simulink model "testRemoteVelEnc"  (Simulink 7.3)
settings: Solver=ode45  SolverMode=SingleTasking  StartTime=0.0  StopTime=inf  FixedStep=0.5  RelTol=1e-3  AbsTol=1e-6
libraries: utility x1
settings Model: Creator=dmedonza  LastModifiedBy=yo
settings DataIOCC: SaveOutput=off  SignalLogging=off  SaveTime=off
settings OptimizationCC: BooleanDataType=off
settings DebuggingCC: SaveWithParameterizedLinksMsg=none  SignalResolutionControl=TryResolveAllWithWarning  SolverPrmCheckMsg=none  MultiTaskDSMMsg=warning  MultiTaskCondExecSysMsg=none  StrictBusMsg=None
settings HardwareCC: TargetUnknown=on
settings RTWCC: TemplateMakefile=grt_vc.tmf  IncludeERTFirstTime=on

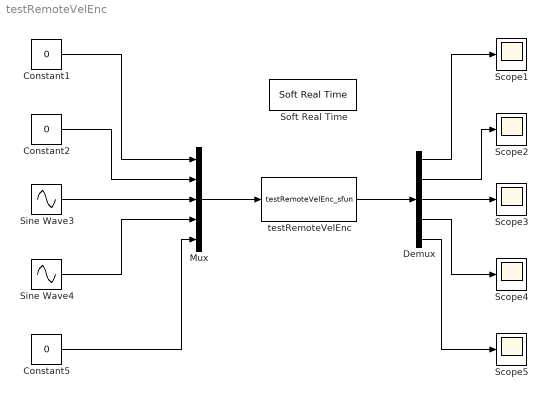
== system testRemoteVelEnc ==
  Constant1 : Constant  Value=0  OutDataType=fixdt(1, 16)  OutScaling=2^0
  Constant2 : Constant  Value=0  OutDataType=fixdt(1, 16)  OutScaling=2^0
  Constant5 : Constant  Value=0  OutDataType=fixdt(1, 16)  OutScaling=2^0
  Demux : Demux  Outputs=5
  Mux : Mux  Inputs=5
  Scope{1..5} (5 alike) : Scope
      Scope1 settings: TimeRange=10  YMin=-1  YMax=1
      Scope2 settings: YMin=-1  YMax=1
      Scope3 settings: YMin=0  YMax=35  SaveName=ScopeData2
      Scope4 settings: YMin=-35  SaveName=ScopeData3
      Scope5 settings: YMin=-70  YMax=0  SaveName=ScopeData4
  Sine Wave3 : Sin  Amplitude=10  Bias=0  Frequency=0.628  Phase=0  Samples=10  SampleTime=0  Offset=0
  Sine Wave4 : Sin  Amplitude=10  Bias=0  Frequency=0.628  Phase=pi  Samples=10  SampleTime=0  Offset=0
  Soft Real Time : utility/Soft Real Time  x=1
  testRemoteVelEnc : S-Function  FunctionName=testRemoteVelEnc_sfun  Parameters='/ravebot' 5  EnableBusSupport=off
      mask Display: image(imread('yarpPipes.png'));
  wires:
  Demux/1 -> Scope1/1
  testRemoteVelEnc/1 -> Demux/1
  Mux/1 -> testRemoteVelEnc/1
  Sine Wave3/1 -> Mux/3
  Constant1/1 -> Mux/1
  Constant2/1 -> Mux/2
  Sine Wave4/1 -> Mux/4
  Constant5/1 -> Mux/5
  Demux/2 -> Scope2/1
  Demux/3 -> Scope3/1
  Demux/4 -> Scope4/1
  Demux/5 -> Scope5/1
